simulink model "spaceShuttleOriginal"  (R2017b)
settings: Solver=FixedStepAuto  StartTime=0.0  StopTime=300  FixedStep=0.08  RelTol=1e-3
undefined symbols (not defined in the file or in its folder): ATTITUDE_ESTIMATE, ATTITUDE_INCREMENT, AUTO_MANUAL_SWITCH, BYPASS, COUNTER, CURRENT_ATTITUDE, DESIRED_ATTITUDE, DESIRED_RATE, INIT_AUTO_MANEUVER, INIT_JET_SELECT, INIT_STATE_ERROR, MANEUVER_HOLD_SW, PRIMARY_JET_COMMAND, RATE_ESTIMATE, UNDESIRED_ACCELERATION_ESTIMATE, VERNIER_JET_COMMAND
libraries: sharedtransform x5, aerolibutil x4, realtime_pacer_lib x1
(part 1 of 3)
settings Model: Creator=raphael  LastModifiedBy=hbourbou

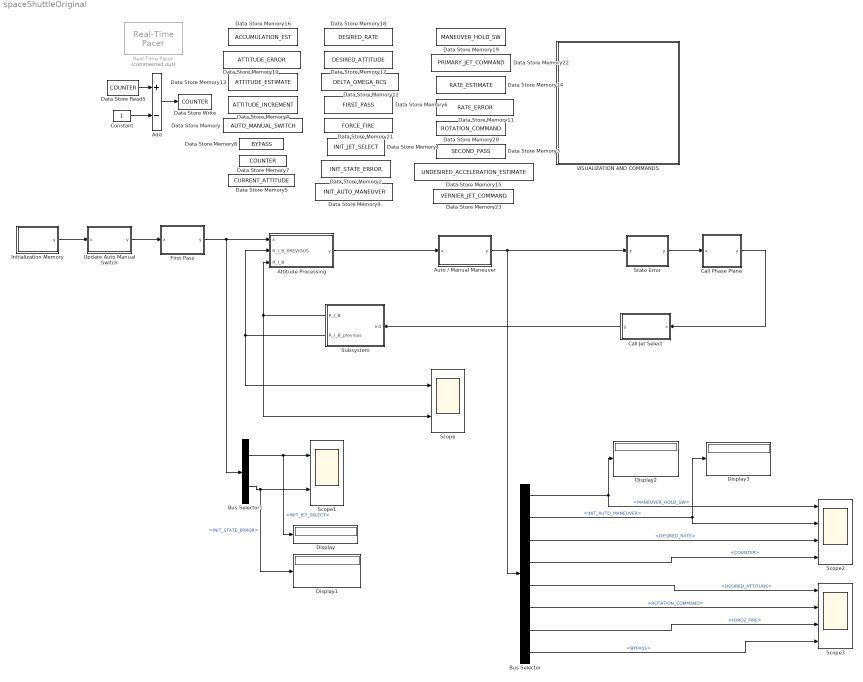
== system spaceShuttleOriginal ==
  Add : Sum  Inputs=+-
  Attitude Processing : Subsystem  Priority=2
  Auto / Manual Maneuver : Subsystem  Priority=2
  Bus Selector : BusSelector  OutputSignals=MANEUVER_HOLD_SW,INIT_AUTO_MANEUVER,DESIRED_RATE,COUNTER,DESIRED_ATTITUDE,ROTATION_COMMAND,FORCE_FIRE,BYPASS
  Bus Selector1 : BusSelector  OutputSignals=INIT_JET_SELECT,INIT_STATE_ERROR
  Call Jet Select : Subsystem  Priority=2
  Call Phase Plane : Subsystem  Priority=2
  Constant : Constant  SampleTime=-1
  Data Store Memory : DataStoreMemory  DataStoreName=AUTO_MANUAL_SWITCH  ReadBeforeWriteMsg=warning  WriteAfterWriteMsg=warning  WriteAfterReadMsg=warning  InitialValue=[0;0]  ShowAdditionalParam=off
  Data Store Memory1 : DataStoreMemory  DataStoreName=INIT_JET_SELECT  ReadBeforeWriteMsg=warning  WriteAfterWriteMsg=warning  WriteAfterReadMsg=warning  ShowAdditionalParam=off
  Data Store Memory10 : DataStoreMemory  DataStoreName=ATTITUDE_ERROR  ReadBeforeWriteMsg=warning  WriteAfterWriteMsg=warning  WriteAfterReadMsg=warning  InitialValue=[0;0;0]  ShowAdditionalParam=off  Dimensions=3
  Data Store Memory11 : DataStoreMemory  DataStoreName=RATE_ERROR  ReadBeforeWriteMsg=warning  WriteAfterWriteMsg=warning  WriteAfterReadMsg=warning  InitialValue=[0;0;0]  ShowAdditionalParam=off  Dimensions=3
  Data Store Memory12 : DataStoreMemory  DataStoreName=DELTA_OMEGA_RCS  ReadBeforeWriteMsg=warning  WriteAfterWriteMsg=warning  WriteAfterReadMsg=warning  InitialValue=[0;0;0]  ShowAdditionalParam=off  Dimensions=3
  Data Store Memory13 : DataStoreMemory  DataStoreName=ATTITUDE_ESTIMATE  ReadBeforeWriteMsg=warning  WriteAfterWriteMsg=warning  WriteAfterReadMsg=warning  InitialValue=[0;0;0]  ShowAdditionalParam=off  Dimensions=3
  Data Store Memory14 : DataStoreMemory  DataStoreName=RATE_ESTIMATE  ReadBeforeWriteMsg=warning  WriteAfterWriteMsg=warning  WriteAfterReadMsg=warning  InitialValue=[0;0;0]  ShowAdditionalParam=off  Dimensions=3
  Data Store Memory15 : DataStoreMemory  DataStoreName=UNDESIRED_ACCELERATION_ESTIMATE  ReadBeforeWriteMsg=warning  WriteAfterWriteMsg=warning  WriteAfterReadMsg=warning  InitialValue=[0;0;0]  ShowAdditionalParam=off  Dimensions=3
  Data Store Memory16 : DataStoreMemory  DataStoreName=ACCUMULATION_EST  ReadBeforeWriteMsg=warning  WriteAfterWriteMsg=warning  WriteAfterReadMsg=warning  InitialValue=[0;0;0]  ShowAdditionalParam=off  Dimensions=3
  Data Store Memory17 : DataStoreMemory  DataStoreName=DESIRED_ATTITUDE  ReadBeforeWriteMsg=warning  WriteAfterWriteMsg=warning  WriteAfterReadMsg=warning  InitialValue=[0;0;0]  ShowAdditionalParam=off  Dimensions=3
  Data Store Memory18 : DataStoreMemory  DataStoreName=DESIRED_RATE  ReadBeforeWriteMsg=warning  WriteAfterWriteMsg=warning  WriteAfterReadMsg=warning  InitialValue=[0;0;0]  ShowAdditionalParam=off  Dimensions=3
  Data Store Memory19 : DataStoreMemory  DataStoreName=MANEUVER_HOLD_SW  ReadBeforeWriteMsg=warning  WriteAfterWriteMsg=warning  WriteAfterReadMsg=warning  InitialValue=[0;0]  ShowAdditionalParam=off  Dimensions=2
  Data Store Memory2 : DataStoreMemory  DataStoreName=INIT_STATE_ERROR  ReadBeforeWriteMsg=warning  WriteAfterWriteMsg=warning  WriteAfterReadMsg=warning  InitialValue=[0;0;0]  ShowAdditionalParam=off  Dimensions=3
  Data Store Memory20 : DataStoreMemory  DataStoreName=ROTATION_COMMAND  ReadBeforeWriteMsg=warning  WriteAfterWriteMsg=warning  WriteAfterReadMsg=warning  InitialValue=[0;0;0]  ShowAdditionalParam=off  Dimensions=3
  Data Store Memory21 : DataStoreMemory  DataStoreName=FORCE_FIRE  ReadBeforeWriteMsg=warning  WriteAfterWriteMsg=warning  WriteAfterReadMsg=warning  InitialValue=[0;0;0]  ShowAdditionalParam=off  Dimensions=3
  Data Store Memory22 : DataStoreMemory  DataStoreName=PRIMARY_JET_COMMAND  ReadBeforeWriteMsg=warning  WriteAfterWriteMsg=warning  WriteAfterReadMsg=warning  InitialValue=[0;0;0;0;0;0;0;0;0;0;0]  ShowAdditionalParam=off  Dimensions=11
  Data Store Memory23 : DataStoreMemory  DataStoreName=VERNIER_JET_COMMAND  ReadBeforeWriteMsg=warning  WriteAfterWriteMsg=warning  WriteAfterReadMsg=warning  InitialValue=[0;0;0;0;0;0]  ShowAdditionalParam=off  Dimensions=6
  Data Store Memory3 : DataStoreMemory  DataStoreName=SECOND_PASS  ReadBeforeWriteMsg=warning  WriteAfterWriteMsg=warning  WriteAfterReadMsg=warning  ShowAdditionalParam=off
  Data Store Memory4 : DataStoreMemory  DataStoreName=ATTITUDE_INCREMENT  ReadBeforeWriteMsg=warning  WriteAfterWriteMsg=warning  WriteAfterReadMsg=warning  InitialValue=[0;0;0]  ShowAdditionalParam=off  Dimensions=3
  Data Store Memory5 : DataStoreMemory  DataStoreName=CURRENT_ATTITUDE  ReadBeforeWriteMsg=warning  WriteAfterWriteMsg=warning  WriteAfterReadMsg=warning  InitialValue=[0;0;0;0]  ShowAdditionalParam=off  Dimensions=4
  Data Store Memory6 : DataStoreMemory  DataStoreName=FIRST_PASS  ReadBeforeWriteMsg=warning  WriteAfterWriteMsg=warning  WriteAfterReadMsg=warning  InitialValue=1  ShowAdditionalParam=off  Dimensions=1
  Data Store Memory7 : DataStoreMemory  DataStoreName=COUNTER  ReadBeforeWriteMsg=warning  WriteAfterWriteMsg=warning  WriteAfterReadMsg=warning  ShowAdditionalParam=off  Dimensions=1
  Data Store Memory8 : DataStoreMemory  DataStoreName=BYPASS  ReadBeforeWriteMsg=warning  WriteAfterWriteMsg=warning  WriteAfterReadMsg=warning  InitialValue=[1;1;1]  ShowAdditionalParam=off  Dimensions=3
  Data Store Memory9 : DataStoreMemory  DataStoreName=INIT_AUTO_MANEUVER  ReadBeforeWriteMsg=warning  WriteAfterWriteMsg=warning  WriteAfterReadMsg=warning  InitialValue=[0]  ShowAdditionalParam=off  Dimensions=1
  Data Store Read5 : DataStoreRead  DataStoreName=COUNTER
  Data Store Write : DataStoreWrite  DataStoreName=COUNTER
  Display{,1..3} (4 alike) : Display
  First Pass : Subsystem  Priority=2
  Initialization Memory : Subsystem
  Real-Time Pacer : realtime_pacer_lib/Real-Time Pacer  Commented=on  simTimePerRealTime=1
  Scope : Scope  NumInputPorts=2
  Scope1 : Scope  NumInputPorts=2
  Scope2 : Scope  NumInputPorts=4
  Scope3 : Scope  NumInputPorts=4
  State Error : Subsystem  Priority=2
  Subsystem : Subsystem
      mask Display: image(imread('spaceShuttle.jpg','jpg'),'center')
  Update Auto Manual Switch : Subsystem  Priority=2
  VISUALIZATION AND COMMANDS : Subsystem
  wires:
  Update Auto Manual Switch/1(y) -> First Pass/1(x)
  First Pass/1(y) -> Bus Selector1/1, Attitude Processing/1(x)
  Data Store Read5/1 -> Add/1
  Constant/1 -> Add/2
  Add/1 -> Data Store Write/1
  Attitude Processing/1(y) -> Auto / Manual Maneuver/1(x)
  Auto / Manual Maneuver/1(y) -> Bus Selector/1, State Error/1(x)
  State Error/1(y) -> Call Phase Plane/1(x)
  Call Phase Plane/1(y) -> Call Jet Select/1(x)
  Call Jet Select/1(y) -> Subsystem/1(In1)
  Subsystem/1(R_I_B) -> Attitude Processing/3(R_I_B), Scope/2
  Subsystem/2(R_I_B_previous) -> Attitude Processing/2(R_I_B_PREVIOUS), Scope/1
  Initialization Memory/1(y) -> Update Auto Manual Switch/1(x)
  Bus Selector/1 -> Display2/1, Scope2/1  "<MANEUVER_HOLD_SW>"
  Bus Selector/2 -> Display3/1, Scope2/2  "<INIT_AUTO_MANEUVER>"
  Bus Selector/3 -> Scope2/3  "<DESIRED_RATE>"
  Bus Selector/4 -> Scope2/4  "<COUNTER>"
  Bus Selector1/1 -> Display/1, Scope1/1  "<INIT_JET_SELECT>"
  Bus Selector1/2 -> Display1/1, Scope1/2  "<INIT_STATE_ERROR>"
  Bus Selector/5 -> Scope3/1  "<DESIRED_ATTITUDE>"
  Bus Selector/6 -> Scope3/2  "<ROTATION_COMMAND>"
  Bus Selector/7 -> Scope3/3  "<FORCE_FIRE>"
  Bus Selector/8 -> Scope3/4  "<BYPASS>"

== system spaceShuttleOriginal/Attitude Processing ==
  x : Inport
  R_I_B_PREVIOUS : Inport  Port=2
  R_I_B : Inport  Port=3
  Data Store Read : DataStoreRead  DataStoreName=SECOND_PASS
  If : If  IfExpression=u1 == 1
  Merge : Merge
  SECOND_PASS == 0 : Subsystem  TreatAsAtomicUnit=on
  SECOND_PASS == 1 : Subsystem  TreatAsAtomicUnit=on
  y : Outport
  wires:
  x/1 -> SECOND_PASS == 0/1(x), SECOND_PASS == 1/1(x)
  Data Store Read/1 -> If/1
  SECOND_PASS == 1/1(y) -> Merge/1
  If/1 -> SECOND_PASS == 1/Action
  If/2 -> SECOND_PASS == 0/Action
  SECOND_PASS == 0/1(y) -> Merge/2
  Merge/1 -> y/1
  R_I_B/1 -> SECOND_PASS == 1/2(R_I_B)
  R_I_B_PREVIOUS/1 -> SECOND_PASS == 1/3(R_I_B1)

== system spaceShuttleOriginal/Auto // Manual Maneuver ==
  x : Inport
  Bus Selector1 : BusSelector  OutputSignals=AUTO_MANUAL_SWITCH
  IF MANUAL : Subsystem  TreatAsAtomicUnit=on
  If : If  IfExpression=u1 == 1
  If AUTO : Subsystem  TreatAsAtomicUnit=on
  Merge : Merge
  Selector : Selector  InputPortWidth=2  IndexOptions=Index vector (dialog)  Indices=[1]  OutputSizes=1
  y : Outport
  wires:
  Selector/1 -> If/1
  If/1 -> If AUTO/Action
  Bus Selector1/1 -> Selector/1  "<AUTO_MANUAL_SWITCH>"
  x/1 -> IF MANUAL/1(x), If AUTO/1(x), Bus Selector1/1
  If/2 -> IF MANUAL/Action
  Merge/1 -> y/1
  IF MANUAL/1(y) -> Merge/2
  If AUTO/1(Out1) -> Merge/1

== system spaceShuttleOriginal/Call Jet Select ==
  x : Inport
  Bus Assignment : BusAssignment  AssignedSignals=INIT_JET_SELECT
  Bus Selector1 : BusSelector  OutputSignals=USER_INPUTS.PRIMARY_VERNIER_SW
  Constant2 : Constant  Value=0
  Data Store Write : DataStoreWrite  DataStoreName=INIT_JET_SELECT
  If : If  IfExpression=u1 == 1
  Merge : Merge
  PRIMARY JETS : Subsystem  TreatAsAtomicUnit=on
  VERNIER JETS : Subsystem  TreatAsAtomicUnit=on
  y : Outport
  wires:
  x/1 -> VERNIER JETS/1(x), PRIMARY JETS/1(In1), Bus Selector1/1
  If/1 -> PRIMARY JETS/Action
  PRIMARY JETS/1(y) -> Merge/1
  If/2 -> VERNIER JETS/Action
  Bus Selector1/1 -> If/1  "<PRIMARY_VERNIER_SW>"
  VERNIER JETS/1(y) -> Merge/2
  Constant2/1 -> Bus Assignment/2, Data Store Write/1
  Merge/1 -> Bus Assignment/1
  Bus Assignment/1 -> y/1

== system spaceShuttleOriginal/Call Phase Plane ==
  x : Inport
  Bus Assignment : BusAssignment  AssignedSignals=ROTATION_COMMAND
  Data Store Write : DataStoreWrite  DataStoreName=ROTATION_COMMAND
  Display : Display
  Get Rotation Pitch : Subsystem
  Get Rotation Roll : Subsystem
  Get Rotation Yaw : Subsystem
  Mux : Mux  Inputs=3
  y : Outport
  wires:
  x/1 -> Get Rotation Roll/1(In1), Bus Assignment/1, Get Rotation Yaw/1(In1), Get Rotation Pitch/1(In1)
  Get Rotation Yaw/1(Out1) -> Mux/3
  Mux/1 -> Display/1, Data Store Write/1, Bus Assignment/2
  Get Rotation Roll/1(Out1) -> Mux/1
  Get Rotation Pitch/1(Out1) -> Mux/2
  Bus Assignment/1 -> y/1

== system spaceShuttleOriginal/First Pass ==
  x : Inport
  Bus Selector : BusSelector  OutputSignals=FIRST_PASS
  If : If  IfExpression=u1 == 1
  If First Pass : Subsystem  TreatAsAtomicUnit=on
  If not first pass : Subsystem  TreatAsAtomicUnit=on
  Merge : Merge
  y : Outport
  wires:
  x/1 -> If not first pass/1(In1), Bus Selector/1, If First Pass/1(In1)
  If not first pass/1(x) -> Merge/2
  If/1 -> If First Pass/Action
  If/2 -> If not first pass/Action
  If First Pass/1(x) -> Merge/1
  Merge/1 -> y/1
  Bus Selector/1 -> If/1  "<FIRST_PASS>"

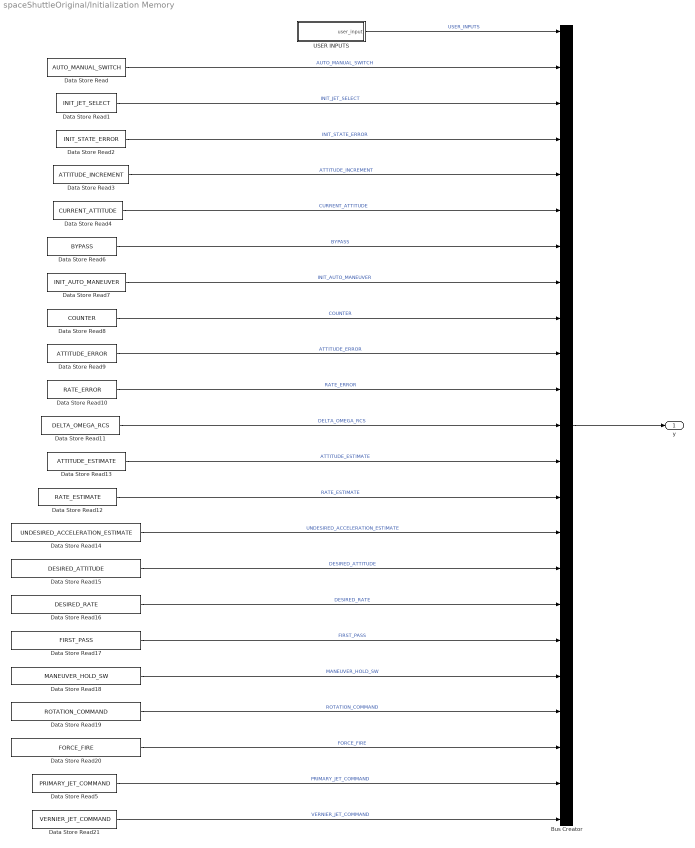
== system spaceShuttleOriginal/Initialization Memory ==
  Bus Creator : BusCreator  Inputs=23
  Data Store Read : DataStoreRead  DataStoreName=AUTO_MANUAL_SWITCH
  Data Store Read1 : DataStoreRead  DataStoreName=INIT_JET_SELECT
  Data Store Read10 : DataStoreRead  DataStoreName=RATE_ERROR
  Data Store Read11 : DataStoreRead  DataStoreName=DELTA_OMEGA_RCS
  Data Store Read12 : DataStoreRead  DataStoreName=RATE_ESTIMATE
  Data Store Read13 : DataStoreRead  DataStoreName=ATTITUDE_ESTIMATE
  Data Store Read14 : DataStoreRead  DataStoreName=UNDESIRED_ACCELERATION_ESTIMATE
  Data Store Read15 : DataStoreRead  DataStoreName=DESIRED_ATTITUDE
  Data Store Read16 : DataStoreRead  DataStoreName=DESIRED_RATE
  Data Store Read17 : DataStoreRead  DataStoreName=FIRST_PASS
  Data Store Read18 : DataStoreRead  DataStoreName=MANEUVER_HOLD_SW
  Data Store Read19 : DataStoreRead  DataStoreName=ROTATION_COMMAND
  Data Store Read2 : DataStoreRead  DataStoreName=INIT_STATE_ERROR
  Data Store Read20 : DataStoreRead  DataStoreName=FORCE_FIRE
  Data Store Read21 : DataStoreRead  DataStoreName=VERNIER_JET_COMMAND
  Data Store Read3 : DataStoreRead  DataStoreName=ATTITUDE_INCREMENT
  Data Store Read4 : DataStoreRead  DataStoreName=CURRENT_ATTITUDE
  Data Store Read5 : DataStoreRead  DataStoreName=PRIMARY_JET_COMMAND
  Data Store Read6 : DataStoreRead  DataStoreName=BYPASS
  Data Store Read7 : DataStoreRead  DataStoreName=INIT_AUTO_MANEUVER
  Data Store Read8 : DataStoreRead  DataStoreName=COUNTER
  Data Store Read9 : DataStoreRead  DataStoreName=ATTITUDE_ERROR
  USER INPUTS : Subsystem  Priority=1
  y : Outport
  wires:
  Data Store Read/1 -> Bus Creator/2  "AUTO_MANUAL_SWITCH"
  Data Store Read1/1 -> Bus Creator/3  "INIT_JET_SELECT"
  Data Store Read2/1 -> Bus Creator/4  "INIT_STATE_ERROR"
  Data Store Read3/1 -> Bus Creator/5  "ATTITUDE_INCREMENT"
  Data Store Read4/1 -> Bus Creator/6  "CURRENT_ATTITUDE"
  Data Store Read6/1 -> Bus Creator/7  "BYPASS"
  Data Store Read7/1 -> Bus Creator/8  "INIT_AUTO_MANEUVER"
  Data Store Read8/1 -> Bus Creator/9  "COUNTER"
  Data Store Read9/1 -> Bus Creator/10  "ATTITUDE_ERROR"
  Data Store Read10/1 -> Bus Creator/11  "RATE_ERROR"
  Data Store Read11/1 -> Bus Creator/12  "DELTA_OMEGA_RCS"
  Data Store Read14/1 -> Bus Creator/15  "UNDESIRED_ACCELERATION_ESTIMATE"
  Data Store Read13/1 -> Bus Creator/13  "ATTITUDE_ESTIMATE"
  Data Store Read12/1 -> Bus Creator/14  "RATE_ESTIMATE"
  Data Store Read15/1 -> Bus Creator/16  "DESIRED_ATTITUDE"
  Data Store Read16/1 -> Bus Creator/17  "DESIRED_RATE"
  Data Store Read17/1 -> Bus Creator/18  "FIRST_PASS"
  Bus Creator/1 -> y/1
  Data Store Read18/1 -> Bus Creator/19  "MANEUVER_HOLD_SW"
  Data Store Read19/1 -> Bus Creator/20  "ROTATION_COMMAND"
  Data Store Read20/1 -> Bus Creator/21  "FORCE_FIRE"
  Data Store Read5/1 -> Bus Creator/22  "PRIMARY_JET_COMMAND"
  USER INPUTS/1(user_input) -> Bus Creator/1  "USER_INPUTS"
  Data Store Read21/1 -> Bus Creator/23  "VERNIER_JET_COMMAND"

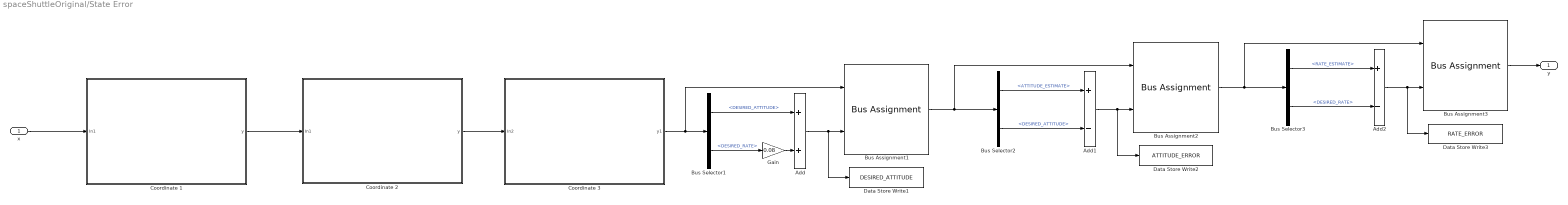
== system spaceShuttleOriginal/State Error ==
  x : Inport
  Add : Sum
  Add1 : Sum  Inputs=+-
  Add2 : Sum  Inputs=+-
  Bus Assignment1 : BusAssignment  AssignedSignals=DESIRED_ATTITUDE
  Bus Assignment2 : BusAssignment  AssignedSignals=ATTITUDE_ERROR
  Bus Assignment3 : BusAssignment  AssignedSignals=RATE_ERROR
  Bus Selector1 : BusSelector  OutputSignals=DESIRED_ATTITUDE,DESIRED_RATE
  Bus Selector2 : BusSelector  OutputSignals=ATTITUDE_ESTIMATE,DESIRED_ATTITUDE
  Bus Selector3 : BusSelector  OutputSignals=RATE_ESTIMATE,DESIRED_RATE
  Coordinate 1 : Subsystem
  Coordinate 2 : Subsystem
  Coordinate 3 : Subsystem
  Data Store Write1 : DataStoreWrite  DataStoreName=DESIRED_ATTITUDE
  Data Store Write2 : DataStoreWrite  DataStoreName=ATTITUDE_ERROR
  Data Store Write3 : DataStoreWrite  DataStoreName=RATE_ERROR
  Gain : Gain  Gain=0.08
  y : Outport
  wires:
  x/1 -> Coordinate 1/1(In1)
  Coordinate 2/1(y) -> Coordinate 3/1(In2)
  Coordinate 1/1(y) -> Coordinate 2/1(In1)
  Bus Assignment1/1 -> Bus Assignment2/1, Bus Selector2/1
  Gain/1 -> Add/2
  Bus Selector2/2 -> Add1/2  "<DESIRED_ATTITUDE>"
  Bus Selector1/1 -> Add/1  "<DESIRED_ATTITUDE>"
  Bus Selector2/1 -> Add1/1  "<ATTITUDE_ESTIMATE>"
  Bus Selector3/2 -> Add2/2  "<DESIRED_RATE>"
  Add1/1 -> Bus Assignment2/2, Data Store Write2/1
  Bus Selector3/1 -> Add2/1  "<RATE_ESTIMATE>"
  Bus Assignment2/1 -> Bus Assignment3/1, Bus Selector3/1
  Bus Assignment3/1 -> y/1
  Add/1 -> Bus Assignment1/2, Data Store Write1/1
  Bus Selector1/2 -> Gain/1  "<DESIRED_RATE>"
  Coordinate 3/1(y1) -> Bus Selector1/1, Bus Assignment1/1
  Add2/1 -> Bus Assignment3/2, Data Store Write3/1

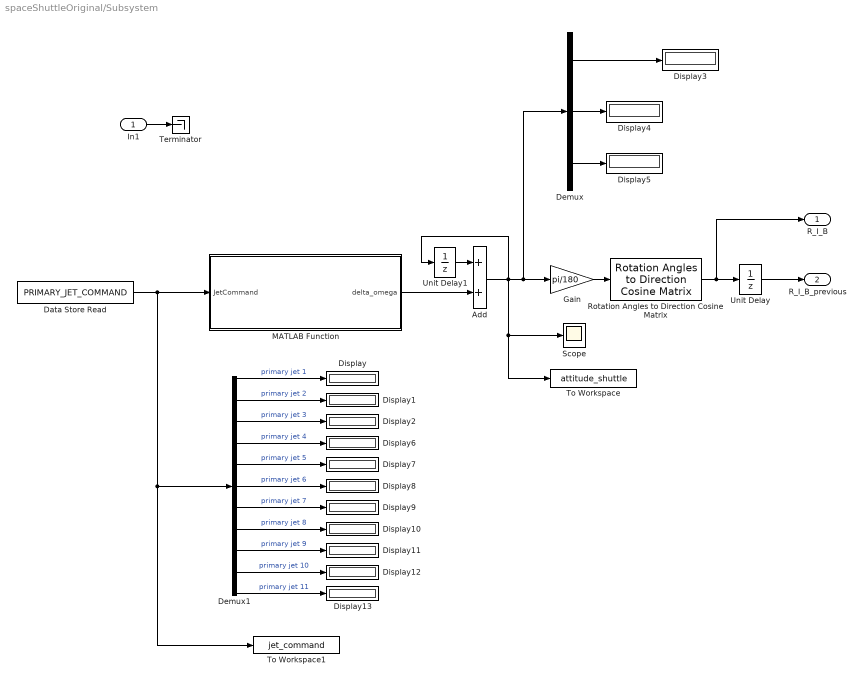
== system spaceShuttleOriginal/Subsystem ==
  In1 : Inport
  Add : Sum
  Data Store Read : DataStoreRead  DataStoreName=PRIMARY_JET_COMMAND
  Demux : Demux  Outputs=3
  Demux1 : Demux  Outputs=11
  Display{,1..13} (14 alike) : Display
  Gain : Gain  Gain=pi/180
  MATLAB Function : MATLAB Function  TreatAsAtomicUnit=on
  Rotation Angles to Direction Cosine Matrix : sharedtransform/Rotation Angles to Direction Cosine Matrix  rotationOrder=XYZ
      settings: SourceProductBaseCode=AE
  Scope : Scope
  Terminator : Terminator
  To Workspace : ToWorkspace  VariableName=attitude_shuttle  SaveFormat=Timeseries  SampleTime=-1
  To Workspace1 : ToWorkspace  VariableName=jet_command  SaveFormat=Timeseries  SampleTime=-1
  Unit Delay : UnitDelay  InitialCondition=eye(3)  SampleTime=-1
  Unit Delay1 : UnitDelay  InitialCondition=[50;50;50]  SampleTime=-1
  R_I_B : Outport
  R_I_B_previous : Outport  Port=2
  wires:
  Gain/1 -> Rotation Angles to Direction Cosine Matrix/1
  Unit Delay1/1 -> Add/1
  Add/1 -> Gain/1, Demux/1, To Workspace/1, Scope/1, Unit Delay1/1
  MATLAB Function/1(delta_omega) -> Add/2
  Demux/3 -> Display5/1
  Demux/2 -> Display4/1
  Demux/1 -> Display3/1
  Demux1/1 -> Display/1  "primary jet 1"
  Demux1/2 -> Display1/1  "primary jet 2"
  Demux1/7 -> Display9/1  "primary jet 7"
  Demux1/6 -> Display8/1  "primary jet 6"
  Demux1/5 -> Display7/1  "primary jet 5"
  Demux1/4 -> Display6/1  "primary jet 4"
  Demux1/3 -> Display2/1  "primary jet 3"
  Demux1/9 -> Display11/1  "primary jet 9"
  Demux1/8 -> Display10/1  "primary jet 8"
  Demux1/10 -> Display12/1  "primary jet 10"
  Demux1/11 -> Display13/1  "primary jet 11"
  Unit Delay/1 -> R_I_B_previous/1
  Rotation Angles to Direction Cosine Matrix/1 -> R_I_B/1, Unit Delay/1
  In1/1 -> Terminator/1
  Data Store Read/1 -> Demux1/1, To Workspace1/1, MATLAB Function/1(JetCommand)

== system spaceShuttleOriginal/Update Auto Manual Switch ==
  x : Inport
  Bus Selector : BusSelector  OutputSignals=RHC_STATE
  Bus Selector1 : BusSelector  OutputSignals=USER_INPUTS
  Dot Product : DotProduct  InputSameDT=on  OutDataTypeStr=Inherit: Inherit via internal rule
  IF RHC : Subsystem  TreatAsAtomicUnit=on
  If : If  IfExpression=u1 ~= 0
  Merge : Merge
  NO RHC : Subsystem  TreatAsAtomicUnit=on
  Sqrt : Sqrt  SaturateOnIntegerOverflow=on
  y : Outport
  wires:
  Dot Product/1 -> Sqrt/1
  If/1 -> IF RHC/Action
  x/1 -> Bus Selector1/1, IF RHC/1(In1), NO RHC/1(In1)
  Bus Selector/1 -> Dot Product/1, Dot Product/2  "<RHC_STATE>"
  If/2 -> NO RHC/Action
  IF RHC/1(x) -> Merge/1
  NO RHC/1(x1) -> Merge/2
  Merge/1 -> y/1
  Sqrt/1 -> If/1
  Bus Selector1/1 -> Bus Selector/1  "<USER_INPUTS>"

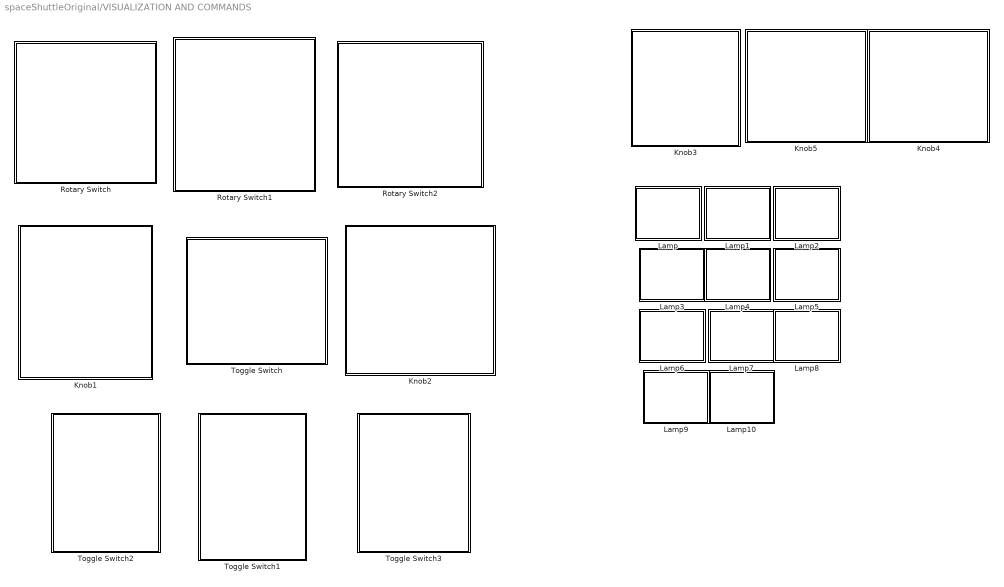
== system spaceShuttleOriginal/VISUALIZATION AND COMMANDS ==
  Knob1 : Subsystem  DialogController=hmiCreateDDGDialog  IsWebBlock=on  mask(MWDashboardBlock){webBlockId=fcc256ec-b885-471c-9536-edbe70c05013, webBlockType=continuousknob, ShowInLibBrowser=on, ShowInitialText=on, HMISrcModelName=spaceShuttleOriginal}
      mask prompts: webBlockId "WebBlock Id"; webBlockType "WebBlock Type"; HMISrcModelName "Source Model"
      mask help: SimulinkHMI:dialogs:ContinuousKnobDialogDesc
      mask Help: helpview([docroot '/mapfiles/simulink.map'], 'hmi_knob')
      mask Display:
      | if strcmp(get_param(bdroot(gcb),'BlockDiagramType'), 'library')
      |     image([(matlabroot) '/toolbox/simulink/hmi/icons/ContinuousKnob.png']);
      | end
  Knob2 : Subsystem  DialogController=hmiCreateDDGDialog  IsWebBlock=on  mask(MWDashboardBlock){webBlockId=8f75210b-2a30-49d8-9c3f-54d330528343, webBlockType=continuousknob, ShowInLibBrowser=on, ShowInitialText=on, HMISrcModelName=spaceShuttleOriginal}
      mask prompts: webBlockId "WebBlock Id"; webBlockType "WebBlock Type"; HMISrcModelName "Source Model"
      mask help: SimulinkHMI:dialogs:ContinuousKnobDialogDesc
      mask Help: helpview([docroot '/mapfiles/simulink.map'], 'hmi_knob')
      mask Display:
      | if strcmp(get_param(bdroot(gcb),'BlockDiagramType'), 'library')
      |     image([(matlabroot) '/toolbox/simulink/hmi/icons/ContinuousKnob.png']);
      | end
  Knob3 : Subsystem  DialogController=hmiCreateDDGDialog  IsWebBlock=on  mask(MWDashboardBlock){webBlockId=1d9576ac-1a07-4627-a000-52538d07e885, webBlockType=continuousknob, ShowInLibBrowser=on, ShowInitialText=on, HMISrcModelName=spaceShuttleOriginal}
      mask prompts: webBlockId "WebBlock Id"; webBlockType "WebBlock Type"; HMISrcModelName "Source Model"
      mask help: SimulinkHMI:dialogs:ContinuousKnobDialogDesc
      mask Help: helpview([docroot '/mapfiles/simulink.map'], 'hmi_knob')
      mask Display:
      | if strcmp(get_param(bdroot(gcb),'BlockDiagramType'), 'library')
      |     image([(matlabroot) '/toolbox/simulink/hmi/icons/ContinuousKnob.png']);
      | end
  Knob4 : Subsystem  DialogController=hmiCreateDDGDialog  IsWebBlock=on  mask(MWDashboardBlock){webBlockId=ba6a8299-7a60-4fd1-b3c4-837f140646ce, webBlockType=continuousknob, ShowInLibBrowser=on, ShowInitialText=on, HMISrcModelName=spaceShuttleOriginal}
      mask prompts: webBlockId "WebBlock Id"; webBlockType "WebBlock Type"; HMISrcModelName "Source Model"
      mask help: SimulinkHMI:dialogs:ContinuousKnobDialogDesc
      mask Help: helpview([docroot '/mapfiles/simulink.map'], 'hmi_knob')
      mask Display:
      | if strcmp(get_param(bdroot(gcb),'BlockDiagramType'), 'library')
      |     image([(matlabroot) '/toolbox/simulink/hmi/icons/ContinuousKnob.png']);
      | end
  Knob5 : Subsystem  DialogController=hmiCreateDDGDialog  IsWebBlock=on  mask(MWDashboardBlock){webBlockId=36d52b40-e662-4d56-9627-14147bf9ee74, webBlockType=continuousknob, ShowInLibBrowser=on, ShowInitialText=on, HMISrcModelName=spaceShuttleOriginal}
      mask prompts: webBlockId "WebBlock Id"; webBlockType "WebBlock Type"; HMISrcModelName "Source Model"
      mask help: SimulinkHMI:dialogs:ContinuousKnobDialogDesc
      mask Help: helpview([docroot '/mapfiles/simulink.map'], 'hmi_knob')
      mask Display:
      | if strcmp(get_param(bdroot(gcb),'BlockDiagramType'), 'library')
      |     image([(matlabroot) '/toolbox/simulink/hmi/icons/ContinuousKnob.png']);
      | end
  Lamp : Subsystem  DialogController=hmiCreateDDGDialog  IsWebBlock=on  mask(MWDashboardBlock){webBlockId=1831b2f3-6b24-4792-bd35-9106f5a9402c, webBlockType=lamp, ShowInLibBrowser=on, ShowInitialText=on, HMISrcModelName=spaceShuttleOriginal}
      mask prompts: webBlockType "WebBlock Type"; HMISrcModelName "Source Model"
      mask help: SimulinkHMI:dialogs:LampDialogDesc
      mask Help: helpview([docroot '/mapfiles/simulink.map'], 'hmi_lamp')
      mask Display:
      | if strcmp(get_param(bdroot(gcb),'BlockDiagramType'), 'library')
      |     image([(matlabroot) '/toolbox/simulink/hmi/icons/Lamp.png']);
      | end
  Lamp1 : Subsystem  DialogController=hmiCreateDDGDialog  IsWebBlock=on  mask(MWDashboardBlock){webBlockId=445b80d1-ef4e-4a60-adf9-cfd209c84993, webBlockType=lamp, ShowInLibBrowser=on, ShowInitialText=on, HMISrcModelName=spaceShuttleOriginal}
      mask prompts: webBlockType "WebBlock Type"; HMISrcModelName "Source Model"
      mask help: SimulinkHMI:dialogs:LampDialogDesc
      mask Help: helpview([docroot '/mapfiles/simulink.map'], 'hmi_lamp')
      mask Display:
      | if strcmp(get_param(bdroot(gcb),'BlockDiagramType'), 'library')
      |     image([(matlabroot) '/toolbox/simulink/hmi/icons/Lamp.png']);
      | end
  Lamp10 : Subsystem  DialogController=hmiCreateDDGDialog  IsWebBlock=on  mask(MWDashboardBlock){webBlockId=5e79d13d-1851-4c1d-ad64-373adbe08a7d, webBlockType=lamp, ShowInLibBrowser=on, ShowInitialText=on, HMISrcModelName=spaceShuttleOriginal}
      mask prompts: webBlockType "WebBlock Type"; HMISrcModelName "Source Model"
      mask help: SimulinkHMI:dialogs:LampDialogDesc
      mask Help: helpview([docroot '/mapfiles/simulink.map'], 'hmi_lamp')
      mask Display:
      | if strcmp(get_param(bdroot(gcb),'BlockDiagramType'), 'library')
      |     image([(matlabroot) '/toolbox/simulink/hmi/icons/Lamp.png']);
      | end
  Lamp2 : Subsystem  DialogController=hmiCreateDDGDialog  IsWebBlock=on  mask(MWDashboardBlock){webBlockId=fe722917-839e-4c17-b303-c27dc3d815a5, webBlockType=lamp, ShowInLibBrowser=on, ShowInitialText=on, HMISrcModelName=spaceShuttleOriginal}
      mask prompts: webBlockType "WebBlock Type"; HMISrcModelName "Source Model"
      mask help: SimulinkHMI:dialogs:LampDialogDesc
      mask Help: helpview([docroot '/mapfiles/simulink.map'], 'hmi_lamp')
      mask Display:
      | if strcmp(get_param(bdroot(gcb),'BlockDiagramType'), 'library')
      |     image([(matlabroot) '/toolbox/simulink/hmi/icons/Lamp.png']);
      | end
  Lamp3 : Subsystem  DialogController=hmiCreateDDGDialog  IsWebBlock=on  mask(MWDashboardBlock){webBlockId=892c30e5-c3e8-4f09-b059-7bca243d068a, webBlockType=lamp, ShowInLibBrowser=on, ShowInitialText=on, HMISrcModelName=spaceShuttleOriginal}
      mask prompts: webBlockType "WebBlock Type"; HMISrcModelName "Source Model"
      mask help: SimulinkHMI:dialogs:LampDialogDesc
      mask Help: helpview([docroot '/mapfiles/simulink.map'], 'hmi_lamp')
      mask Display:
      | if strcmp(get_param(bdroot(gcb),'BlockDiagramType'), 'library')
      |     image([(matlabroot) '/toolbox/simulink/hmi/icons/Lamp.png']);
      | end
  Lamp4 : Subsystem  DialogController=hmiCreateDDGDialog  IsWebBlock=on  mask(MWDashboardBlock){webBlockId=c806c832-793b-4743-9fcd-4b551699f67b, webBlockType=lamp, ShowInLibBrowser=on, ShowInitialText=on, HMISrcModelName=spaceShuttleOriginal}
      mask prompts: webBlockType "WebBlock Type"; HMISrcModelName "Source Model"
      mask help: SimulinkHMI:dialogs:LampDialogDesc
      mask Help: helpview([docroot '/mapfiles/simulink.map'], 'hmi_lamp')
      mask Display:
      | if strcmp(get_param(bdroot(gcb),'BlockDiagramType'), 'library')
      |     image([(matlabroot) '/toolbox/simulink/hmi/icons/Lamp.png']);
      | end
  Lamp5 : Subsystem  DialogController=hmiCreateDDGDialog  IsWebBlock=on  mask(MWDashboardBlock){webBlockId=98e8761d-c632-4f86-92e2-3e19c3b791e9, webBlockType=lamp, ShowInLibBrowser=on, ShowInitialText=on, HMISrcModelName=spaceShuttleOriginal}
      mask prompts: webBlockType "WebBlock Type"; HMISrcModelName "Source Model"
      mask help: SimulinkHMI:dialogs:LampDialogDesc
      mask Help: helpview([docroot '/mapfiles/simulink.map'], 'hmi_lamp')
      mask Display:
      | if strcmp(get_param(bdroot(gcb),'BlockDiagramType'), 'library')
      |     image([(matlabroot) '/toolbox/simulink/hmi/icons/Lamp.png']);
      | end
  Lamp6 : Subsystem  DialogController=hmiCreateDDGDialog  IsWebBlock=on  mask(MWDashboardBlock){webBlockId=f963022c-aea4-457b-adfc-b083e719e9f5, webBlockType=lamp, ShowInLibBrowser=on, ShowInitialText=on, HMISrcModelName=spaceShuttleOriginal}
      mask prompts: webBlockType "WebBlock Type"; HMISrcModelName "Source Model"
      mask help: SimulinkHMI:dialogs:LampDialogDesc
      mask Help: helpview([docroot '/mapfiles/simulink.map'], 'hmi_lamp')
      mask Display:
      | if strcmp(get_param(bdroot(gcb),'BlockDiagramType'), 'library')
      |     image([(matlabroot) '/toolbox/simulink/hmi/icons/Lamp.png']);
      | end
  Lamp7 : Subsystem  DialogController=hmiCreateDDGDialog  IsWebBlock=on  mask(MWDashboardBlock){webBlockId=74668ae3-2b37-4bc0-806e-989ea60bf3f3, webBlockType=lamp, ShowInLibBrowser=on, ShowInitialText=on, HMISrcModelName=spaceShuttleOriginal}
      mask prompts: webBlockType "WebBlock Type"; HMISrcModelName "Source Model"
      mask help: SimulinkHMI:dialogs:LampDialogDesc
      mask Help: helpview([docroot '/mapfiles/simulink.map'], 'hmi_lamp')
      mask Display:
      | if strcmp(get_param(bdroot(gcb),'BlockDiagramType'), 'library')
      |     image([(matlabroot) '/toolbox/simulink/hmi/icons/Lamp.png']);
      | end
  Lamp8 : Subsystem  DialogController=hmiCreateDDGDialog  IsWebBlock=on  mask(MWDashboardBlock){webBlockId=a86ecc11-9b5f-486c-a116-6a169a848fb0, webBlockType=lamp, ShowInLibBrowser=on, ShowInitialText=on, HMISrcModelName=spaceShuttleOriginal}
      mask prompts: webBlockType "WebBlock Type"; HMISrcModelName "Source Model"
      mask help: SimulinkHMI:dialogs:LampDialogDesc
      mask Help: helpview([docroot '/mapfiles/simulink.map'], 'hmi_lamp')
      mask Display:
      | if strcmp(get_param(bdroot(gcb),'BlockDiagramType'), 'library')
      |     image([(matlabroot) '/toolbox/simulink/hmi/icons/Lamp.png']);
      | end
  Lamp9 : Subsystem  DialogController=hmiCreateDDGDialog  IsWebBlock=on  mask(MWDashboardBlock){webBlockId=f4dbbe1a-4ec4-452b-b5cc-403f6e1bd4d4, webBlockType=lamp, ShowInLibBrowser=on, ShowInitialText=on, HMISrcModelName=spaceShuttleOriginal}
      mask prompts: webBlockType "WebBlock Type"; HMISrcModelName "Source Model"
      mask help: SimulinkHMI:dialogs:LampDialogDesc
      mask Help: helpview([docroot '/mapfiles/simulink.map'], 'hmi_lamp')
      mask Display:
      | if strcmp(get_param(bdroot(gcb),'BlockDiagramType'), 'library')
      |     image([(matlabroot) '/toolbox/simulink/hmi/icons/Lamp.png']);
      | end
  Rotary Switch : Subsystem  DialogController=hmiCreateDDGDialog  IsWebBlock=on  mask(MWDashboardBlock){webBlockId=aad051ce-0605-48d0-815b-93b49174babb, webBlockType=discreteknob, ShowInLibBrowser=on, ShowInitialText=on, HMISrcModelName=spaceShuttleOriginal}
      mask prompts: webBlockId "WebBlock Id"; webBlockType "WebBlock Type"; HMISrcModelName "Source Model"
      mask help: SimulinkHMI:dialogs:DiscreteKnobDialogDesc
      mask Help: helpview([docroot '/mapfiles/simulink.map'], 'hmi_rotary_switch')
      mask Display:
      | model = bdroot(gcb);
      | if strcmp(get_param(model,'BlockDiagramType'), 'library')
      |     image([(matlabroot) '/toolbox/simulink/hmi/icons/DiscreteKnob.png']);
      | end
  Rotary Switch1 : Subsystem  DialogController=hmiCreateDDGDialog  IsWebBlock=on  mask(MWDashboardBlock){webBlockId=d0caed68-568e-4dc9-8d97-a2c88f43b8a4, webBlockType=discreteknob, ShowInLibBrowser=on, ShowInitialText=on, HMISrcModelName=spaceShuttleOriginal}
      mask prompts: webBlockId "WebBlock Id"; webBlockType "WebBlock Type"; HMISrcModelName "Source Model"
      mask help: SimulinkHMI:dialogs:DiscreteKnobDialogDesc
      mask Help: helpview([docroot '/mapfiles/simulink.map'], 'hmi_rotary_switch')
      mask Display:
      | model = bdroot(gcb);
      | if strcmp(get_param(model,'BlockDiagramType'), 'library')
      |     image([(matlabroot) '/toolbox/simulink/hmi/icons/DiscreteKnob.png']);
      | end
  Rotary Switch2 : Subsystem  DialogController=hmiCreateDDGDialog  IsWebBlock=on  mask(MWDashboardBlock){webBlockId=1c4c8ede-caaf-4351-9b32-2d96b9d3b069, webBlockType=discreteknob, ShowInLibBrowser=on, ShowInitialText=on, HMISrcModelName=spaceShuttleOriginal}
      mask prompts: webBlockId "WebBlock Id"; webBlockType "WebBlock Type"; HMISrcModelName "Source Model"
      mask help: SimulinkHMI:dialogs:DiscreteKnobDialogDesc
      mask Help: helpview([docroot '/mapfiles/simulink.map'], 'hmi_rotary_switch')
      mask Display:
      | model = bdroot(gcb);
      | if strcmp(get_param(model,'BlockDiagramType'), 'library')
      |     image([(matlabroot) '/toolbox/simulink/hmi/icons/DiscreteKnob.png']);
      | end
  Toggle Switch : Subsystem  DialogController=hmiCreateDDGDialog  IsWebBlock=on  mask(MWDashboardBlock){webBlockId=a1feb33e-c936-40cb-b89a-58db8a7ab2ae, webBlockType=toggleswitch, ShowInLibBrowser=on, ShowInitialText=on, HMISrcModelName=spaceShuttleOriginal}
      mask prompts: webBlockId "WebBlock Id"; webBlockType "WebBlock Type"; HMISrcModelName "Source Model"
      mask help: SimulinkHMI:dialogs:SwitchDialogDesc
      mask Help: helpview([docroot '/mapfiles/simulink.map'], 'hmi_toggle_switch')
      mask Display:
      | if strcmp(get_param(bdroot(gcb),'BlockDiagramType'), 'library')
      |     image([(matlabroot) '/toolbox/simulink/hmi/icons/ToggleSwitch.png']);
      | end
  Toggle Switch1 : Subsystem  DialogController=hmiCreateDDGDialog  IsWebBlock=on  mask(MWDashboardBlock){webBlockId=632d40ef-ab94-416f-9446-e5cd2c645a87, webBlockType=toggleswitch, ShowInLibBrowser=on, ShowInitialText=on, HMISrcModelName=spaceShuttleOriginal}
      mask prompts: webBlockId "WebBlock Id"; webBlockType "WebBlock Type"; HMISrcModelName "Source Model"
      mask help: SimulinkHMI:dialogs:SwitchDialogDesc
      mask Help: helpview([docroot '/mapfiles/simulink.map'], 'hmi_toggle_switch')
      mask Display:
      | if strcmp(get_param(bdroot(gcb),'BlockDiagramType'), 'library')
      |     image([(matlabroot) '/toolbox/simulink/hmi/icons/ToggleSwitch.png']);
      | end
  Toggle Switch2 : Subsystem  DialogController=hmiCreateDDGDialog  IsWebBlock=on  mask(MWDashboardBlock){webBlockId=c411ff4e-efdd-44a4-8e84-bf7aad950407, webBlockType=toggleswitch, ShowInLibBrowser=on, ShowInitialText=on, HMISrcModelName=spaceShuttleOriginal}
      mask prompts: webBlockId "WebBlock Id"; webBlockType "WebBlock Type"; HMISrcModelName "Source Model"
      mask help: SimulinkHMI:dialogs:SwitchDialogDesc
      mask Help: helpview([docroot '/mapfiles/simulink.map'], 'hmi_toggle_switch')
      mask Display:
      | if strcmp(get_param(bdroot(gcb),'BlockDiagramType'), 'library')
      |     image([(matlabroot) '/toolbox/simulink/hmi/icons/ToggleSwitch.png']);
      | end
  Toggle Switch3 : Subsystem  DialogController=hmiCreateDDGDialog  IsWebBlock=on  mask(MWDashboardBlock){webBlockId=72f03ffd-cacb-422d-91db-5f40b9d6549d, webBlockType=toggleswitch, ShowInLibBrowser=on, ShowInitialText=on, HMISrcModelName=spaceShuttleOriginal}
      mask prompts: webBlockId "WebBlock Id"; webBlockType "WebBlock Type"; HMISrcModelName "Source Model"
      mask help: SimulinkHMI:dialogs:SwitchDialogDesc
      mask Help: helpview([docroot '/mapfiles/simulink.map'], 'hmi_toggle_switch')
      mask Display:
      | if strcmp(get_param(bdroot(gcb),'BlockDiagramType'), 'library')
      |     image([(matlabroot) '/toolbox/simulink/hmi/icons/ToggleSwitch.png']);
      | end

== system spaceShuttleOriginal/Attitude Processing/SECOND_PASS == 0 ==
  x : Inport
  Action Port : ActionPort  ActionType=else
  Bus Assignment1 : BusAssignment  AssignedSignals=ATTITUDE_INCREMENT,CURRENT_ATTITUDE,ATTITUDE_ESTIMATE,RATE_ESTIMATE,UNDESIRED_ACCELERATION_ESTIMATE
  Constant2 : Constant
  Data Store Read : DataStoreRead  DataStoreName=ATTITUDE_INCREMENT
  Data Store Read1 : DataStoreRead  DataStoreName=CURRENT_ATTITUDE
  Data Store Read2 : DataStoreRead  DataStoreName=RATE_ESTIMATE
  Data Store Read3 : DataStoreRead  DataStoreName=ATTITUDE_ESTIMATE
  Data Store Read4 : DataStoreRead  DataStoreName=UNDESIRED_ACCELERATION_ESTIMATE
  Data Store Write1 : DataStoreWrite  DataStoreName=SECOND_PASS
  y : Outport
  wires:
  Constant2/1 -> Data Store Write1/1
  x/1 -> Bus Assignment1/1
  Bus Assignment1/1 -> y/1
  Data Store Read/1 -> Bus Assignment1/2
  Data Store Read1/1 -> Bus Assignment1/3
  Data Store Read3/1 -> Bus Assignment1/4
  Data Store Read2/1 -> Bus Assignment1/5
  Data Store Read4/1 -> Bus Assignment1/6

== system spaceShuttleOriginal/Attitude Processing/SECOND_PASS == 1 ==
  x : Inport
  R_I_B : Inport  Port=2
  R_I_B1 : Inport  Port=3
  Action Port : ActionPort  ActionType=then
  ATTITUDE PROCESSOR : Subsystem
  Bus Assignment : BusAssignment  AssignedSignals=ATTITUDE_INCREMENT,CURRENT_ATTITUDE,ATTITUDE_ESTIMATE,RATE_ESTIMATE,UNDESIRED_ACCELERATION_ESTIMATE
  Constant2 : Constant  Value=0
  Data Store Write1 : DataStoreWrite  DataStoreName=SECOND_PASS
  Data Store Write2 : DataStoreWrite  DataStoreName=CURRENT_ATTITUDE
  Data Store Write3 : DataStoreWrite  DataStoreName=ATTITUDE_INCREMENT
  Data Store Write4 : DataStoreWrite  DataStoreName=ATTITUDE_ESTIMATE
  Data Store Write5 : DataStoreWrite  DataStoreName=RATE_ESTIMATE
  Data Store Write6 : DataStoreWrite  DataStoreName=UNDESIRED_ACCELERATION_ESTIMATE
  State Estimator Part I : Subsystem
  y : Outport
  wires:
  Bus Assignment/1 -> y/1
  Constant2/1 -> Data Store Write1/1
  ATTITUDE PROCESSOR/1(CURRENT ATTITUDE) -> State Estimator Part I/1(CURRENT_ATTITUDE), Bus Assignment/3, Data Store Write2/1
  ATTITUDE PROCESSOR/2(ATTITUDE INCREMENT) -> Bus Assignment/2, Data Store Write3/1
  R_I_B/1 -> ATTITUDE PROCESSOR/1(R_I_B)
  R_I_B1/1 -> ATTITUDE PROCESSOR/2(R_I_B_PREVIOUS)
  x/1 -> Bus Assignment/1
  State Estimator Part I/1(ATTITUDE_ESTIMATE) -> Bus Assignment/4, Data Store Write4/1
  State Estimator Part I/2(RATE_ESTIMATE) -> Bus Assignment/5, Data Store Write5/1
  State Estimator Part I/3(UNDESIRED_ACCELERATION_ESTIMATE) -> Bus Assignment/6, Data Store Write6/1

== system spaceShuttleOriginal/Auto // Manual Maneuver/IF MANUAL ==
  x : Inport
  Action Port : ActionPort  ActionType=else
  MANUAL MANEUVER MODULE : Subsystem
  y : Outport
  wires:
  x/1 -> MANUAL MANEUVER MODULE/1(In1)
  MANUAL MANEUVER MODULE/1(Out1) -> y/1

== system spaceShuttleOriginal/Auto // Manual Maneuver/If AUTO ==
  x : Inport
  Action Port : ActionPort  ActionType=then
  Bus Selector1 : BusSelector  OutputSignals=AUTO_MANUAL_SWITCH
  Bus Selector2 : BusSelector  OutputSignals=COUNTER
  COUNTER ~=0 : Subsystem  TreatAsAtomicUnit=on
  IF COUNTER=0 : Subsystem  TreatAsAtomicUnit=on
  IF OLD=AUTO : Subsystem  TreatAsAtomicUnit=on
  IF OLD=MANUAL : Subsystem  TreatAsAtomicUnit=on
  If : If  IfExpression=u1 == 0
  If1 : If  IfExpression=u1 == 0
  Merge : Merge
  Merge1 : Merge
  Selector : Selector  InputPortWidth=2  IndexOptions=Index vector (dialog)  Indices=[2]  OutputSizes=1
  Out1 : Outport
  wires:
  Bus Selector1/1 -> Selector/1  "<AUTO_MANUAL_SWITCH>"
  If/1 -> IF OLD=MANUAL/Action
  x/1 -> IF OLD=AUTO/1(In1), IF OLD=MANUAL/1(In1), Bus Selector1/1
  Merge/1 -> IF COUNTER=0/1(In2), COUNTER ~=0/1(In1), Bus Selector2/1
  If1/1 -> IF COUNTER=0/Action
  IF OLD=MANUAL/1(Out1) -> Merge/1
  IF OLD=AUTO/1(Out1) -> Merge/2
  If/2 -> IF OLD=AUTO/Action
  If1/2 -> COUNTER ~=0/Action
  COUNTER ~=0/1(Out1) -> Merge1/2
  Bus Selector2/1 -> If1/1  "<COUNTER>"
  Merge1/1 -> Out1/1
  IF COUNTER=0/1(Out1) -> Merge1/1
  Selector/1 -> If/1

== system spaceShuttleOriginal/Call Jet Select/PRIMARY JETS ==
  In1 : Inport
  Action Port : ActionPort  ActionType=then
  Bus Assignment : BusAssignment  AssignedSignals=PRIMARY_JET_COMMAND,VERNIER_JET_COMMAND
  Bus Selector : BusSelector  OutputSignals=ROTATION_COMMAND,USER_INPUTS.PITCH_HI_LOW_SW,USER_INPUTS.NO_PLUS_Z_JETS,USER_INPUTS.PITCH_TAIL_NOSE_SW,USER_INPUTS.YAW_HI_LOW_SW,USER_INPUTS.YAW_TAIL_NOSE_SW
  Constant{,1..3} (4 alike) : Constant  Value=0
  Data Store Write : DataStoreWrite  DataStoreName=PRIMARY_JET_COMMAND
  Data Store Write1 : DataStoreWrite  DataStoreName=VERNIER_JET_COMMAND
  MATLAB Function : MATLAB Function  TreatAsAtomicUnit=on
  Mux : Mux  Inputs=3
  Mux1 : Mux  Inputs=6
  y : Outport
  wires:
  Bus Selector/4 -> MATLAB Function/5(PITCH_TAIL_NOSE_SW)  "<PITCH_TAIL_NOSE_SW>"
  Mux/1 -> MATLAB Function/1(compensationCommand)
  Bus Selector/5 -> MATLAB Function/6(YAW_HI_LOW_SW)  "<YAW_HI_LOW_SW>"
  Bus Selector/6 -> MATLAB Function/7(YAW_TAIL_NOSE_SW)  "<YAW_TAIL_NOSE_SW>"
  Bus Selector/3 -> MATLAB Function/4(NO_PLUS_Z_JETS)  "<NO_PLUS_Z_JETS>"
  Bus Selector/1 -> MATLAB Function/2(rotationCommand)  "<ROTATION_COMMAND>"
  In1/1 -> Bus Selector/1, Bus Assignment/1
  MATLAB Function/1(primaryJetCommand) -> Bus Assignment/2, Data Store Write/1
  Constant2/1 -> Mux/3
  Bus Selector/2 -> MATLAB Function/3(PITCH_HI_LOW_SW)  "<PITCH_HI_LOW_SW>"
  Bus Assignment/1 -> y/1
  Constant1/1 -> Mux/2
  Constant/1 -> Mux/1
  Constant3/1 -> Mux1/6, Mux1/5, Mux1/4, Mux1/1, Mux1/2, Mux1/3
  Mux1/1 -> Bus Assignment/3, Data Store Write1/1

== system spaceShuttleOriginal/Call Jet Select/VERNIER JETS ==
  x : Inport
  Action Port : ActionPort  ActionType=else
  Bus Assignment : BusAssignment  AssignedSignals=VERNIER_JET_COMMAND,PRIMARY_JET_COMMAND
  Constant : Constant  Value=0
  Data Store Write : DataStoreWrite  DataStoreName=PRIMARY_JET_COMMAND
  Data Store Write1 : DataStoreWrite  DataStoreName=VERNIER_JET_COMMAND
  MATLAB Function : MATLAB Function  TreatAsAtomicUnit=on
  Mux : Mux  Inputs=11
  y : Outport
  wires:
  Bus Assignment/1 -> y/1
  Mux/1 -> Bus Assignment/3, Data Store Write/1
  x/1 -> Bus Assignment/1
  Constant/1 -> Mux/2, Mux/1, Mux/3, Mux/4, Mux/5, Mux/11, Mux/10, Mux/9, Mux/8, Mux/7, Mux/6
  MATLAB Function/1(vernierJetCommand) -> Bus Assignment/2, Data Store Write1/1

== system spaceShuttleOriginal/Call Phase Plane/Get Rotation Pitch ==
  In1 : Inport
  Bus Selector : BusSelector  OutputSignals=USER_INPUTS.PRIMARY_VERNIER_SW,UNDESIRED_ACCELERATION_ESTIMATE,USER_INPUTS.DEADBAND,ATTITUDE_ERROR,RATE_ERROR,ROTATION_COMMAND,USER_INPUTS.RATE_LIMIT,BYPASS,FORCE_FIRE
  Constant : Constant  Value=2
  Constant1 : Constant  Value=2
  Constant2 : Constant  Value=2
  Display1 : Display
  MATLAB Function : MATLAB Function  TreatAsAtomicUnit=on
  MATLAB Function1 : MATLAB Function  TreatAsAtomicUnit=on
  MATLAB Function2 : MATLAB Function  TreatAsAtomicUnit=on
  Out1 : Outport
  wires:
  MATLAB Function2/1(command) -> Out1/1
  Constant/1 -> MATLAB Function/1(n)
  MATLAB Function/1(S) -> MATLAB Function1/2(S), MATLAB Function2/3(S)
  Bus Selector/8 -> MATLAB Function2/5(BYPASS)  "<BYPASS>"
  MATLAB Function1/1(index) -> Display1/1, MATLAB Function2/2(index)
  Constant1/1 -> MATLAB Function2/1(n)
  Bus Selector/9 -> MATLAB Function2/9(forceFire)  "<FORCE_FIRE>"
  Constant2/1 -> MATLAB Function1/1(n)
  Bus Selector/7 -> MATLAB Function2/8(rateLimit), MATLAB Function/8(rateLimit)  "<RATE_LIMIT>"
  In1/1 -> Bus Selector/1
  Bus Selector/6 -> MATLAB Function2/6(RC), MATLAB Function/7(rotationCommandn)  "<ROTATION_COMMAND>"
  Bus Selector/5 -> MATLAB Function1/4(we), MATLAB Function2/7(rate_error), MATLAB Function/6(rate_error)  "<RATE_ERROR>"
  Bus Selector/4 -> MATLAB Function1/3(theta_e), MATLAB Function/5(attitude_error)  "<ATTITUDE_ERROR>"
  Bus Selector/3 -> MATLAB Function/4(DB)  "<DEADBAND>"
  Bus Selector/2 -> MATLAB Function1/5(undesired_acc), MATLAB Function/3(undesired_acc)  "<UNDESIRED_ACCELERATION_ESTIMATE>"
  Bus Selector/1 -> MATLAB Function2/4(vernier_sw), MATLAB Function/2(vernier_sw)  "<PRIMARY_VERNIER_SW>"

== system spaceShuttleOriginal/Call Phase Plane/Get Rotation Roll ==
  In1 : Inport
  Bus Selector : BusSelector  OutputSignals=USER_INPUTS.PRIMARY_VERNIER_SW,UNDESIRED_ACCELERATION_ESTIMATE,USER_INPUTS.DEADBAND,ATTITUDE_ERROR,RATE_ERROR,ROTATION_COMMAND,USER_INPUTS.RATE_LIMIT,BYPASS,FORCE_FIRE
  Constant : Constant
  Constant1 : Constant
  Constant2 : Constant
  Display1 : Display
  MATLAB Function : MATLAB Function  TreatAsAtomicUnit=on
  MATLAB Function1 : MATLAB Function  TreatAsAtomicUnit=on
  MATLAB Function2 : MATLAB Function  TreatAsAtomicUnit=on
  Out1 : Outport
  wires:
  MATLAB Function2/1(command) -> Out1/1
  Constant/1 -> MATLAB Function/1(n)
  MATLAB Function/1(S) -> MATLAB Function1/2(S), MATLAB Function2/3(S)
  Bus Selector/8 -> MATLAB Function2/5(BYPASS)  "<BYPASS>"
  MATLAB Function1/1(index) -> Display1/1, MATLAB Function2/2(index)
  Constant1/1 -> MATLAB Function2/1(n)
  Bus Selector/9 -> MATLAB Function2/9(forceFire)  "<FORCE_FIRE>"
  Constant2/1 -> MATLAB Function1/1(n)
  Bus Selector/7 -> MATLAB Function2/8(rateLimit), MATLAB Function/8(rateLimit)  "<RATE_LIMIT>"
  In1/1 -> Bus Selector/1
  Bus Selector/6 -> MATLAB Function2/6(RC), MATLAB Function/7(rotationCommandn)  "<ROTATION_COMMAND>"
  Bus Selector/5 -> MATLAB Function1/4(we), MATLAB Function2/7(rate_error), MATLAB Function/6(rate_error)  "<RATE_ERROR>"
  Bus Selector/4 -> MATLAB Function1/3(theta_e), MATLAB Function/5(attitude_error)  "<ATTITUDE_ERROR>"
  Bus Selector/3 -> MATLAB Function/4(DB)  "<DEADBAND>"
  Bus Selector/2 -> MATLAB Function1/5(undesired_acc), MATLAB Function/3(undesired_acc)  "<UNDESIRED_ACCELERATION_ESTIMATE>"
  Bus Selector/1 -> MATLAB Function2/4(vernier_sw), MATLAB Function/2(vernier_sw)  "<PRIMARY_VERNIER_SW>"

== system spaceShuttleOriginal/Call Phase Plane/Get Rotation Yaw ==
  In1 : Inport
  Bus Selector : BusSelector  OutputSignals=USER_INPUTS.PRIMARY_VERNIER_SW,UNDESIRED_ACCELERATION_ESTIMATE,USER_INPUTS.DEADBAND,ATTITUDE_ERROR,RATE_ERROR,ROTATION_COMMAND,USER_INPUTS.RATE_LIMIT,BYPASS,FORCE_FIRE
  Constant : Constant  Value=3
  Constant1 : Constant  Value=3
  Constant2 : Constant  Value=3
  Display1 : Display
  MATLAB Function : MATLAB Function  TreatAsAtomicUnit=on
  MATLAB Function1 : MATLAB Function  TreatAsAtomicUnit=on
  MATLAB Function2 : MATLAB Function  TreatAsAtomicUnit=on
  Out1 : Outport
  wires:
  MATLAB Function2/1(command) -> Out1/1
  Constant/1 -> MATLAB Function/1(n)
  MATLAB Function/1(S) -> MATLAB Function1/2(S), MATLAB Function2/3(S)
  Bus Selector/8 -> MATLAB Function2/5(BYPASS)  "<BYPASS>"
  MATLAB Function1/1(index) -> Display1/1, MATLAB Function2/2(index)
  Constant1/1 -> MATLAB Function2/1(n)
  Bus Selector/9 -> MATLAB Function2/9(forceFire)  "<FORCE_FIRE>"
  Constant2/1 -> MATLAB Function1/1(n)
  Bus Selector/7 -> MATLAB Function2/8(rateLimit), MATLAB Function/8(rateLimit)  "<RATE_LIMIT>"
  In1/1 -> Bus Selector/1
  Bus Selector/6 -> MATLAB Function2/6(RC), MATLAB Function/7(rotationCommandn)  "<ROTATION_COMMAND>"
  Bus Selector/5 -> MATLAB Function1/4(we), MATLAB Function2/7(rate_error), MATLAB Function/6(rate_error)  "<RATE_ERROR>"
  Bus Selector/4 -> MATLAB Function1/3(theta_e), MATLAB Function/5(attitude_error)  "<ATTITUDE_ERROR>"
  Bus Selector/3 -> MATLAB Function/4(DB)  "<DEADBAND>"
  Bus Selector/2 -> MATLAB Function1/5(undesired_acc), MATLAB Function/3(undesired_acc)  "<UNDESIRED_ACCELERATION_ESTIMATE>"
  Bus Selector/1 -> MATLAB Function2/4(vernier_sw), MATLAB Function/2(vernier_sw)  "<PRIMARY_VERNIER_SW>"

== system spaceShuttleOriginal/First Pass/If First Pass ==
  In1 : Inport
  Action Port : ActionPort  ActionType=then
  AUTO : Subsystem  TreatAsAtomicUnit=on
  Bus Assignment : BusAssignment  AssignedSignals=INIT_JET_SELECT
  Bus Selector : BusSelector  OutputSignals=AUTO_MANUAL_SWITCH
  Constant2 : Constant
  Data Store Write1 : DataStoreWrite  DataStoreName=INIT_JET_SELECT
  If : If  IfExpression=u1 == 0
  MANUAL : Subsystem  TreatAsAtomicUnit=on
  Merge : Merge
  Selector : Selector  InputPortWidth=2  IndexOptions=Index vector (dialog)  Indices=[1]  OutputSizes=1
  x : Outport
  wires:
  In1/1 -> Bus Assignment/1
  Bus Assignment/1 -> AUTO/1(In2), MANUAL/1(In1), Bus Selector/1
  Constant2/1 -> Bus Assignment/2, Data Store Write1/1
  Bus Selector/1 -> Selector/1  "<AUTO_MANUAL_SWITCH>"
  If/1 -> MANUAL/Action
  If/2 -> AUTO/Action
  MANUAL/1(x) -> Merge/1
  Merge/1 -> x/1
  Selector/1 -> If/1
  AUTO/1(x1) -> Merge/2

== system spaceShuttleOriginal/First Pass/If not first pass ==
  In1 : Inport
  Action Port : ActionPort  ActionType=else
  Bus Assignment : BusAssignment  AssignedSignals=INIT_JET_SELECT,INIT_STATE_ERROR
  Data Store Read : DataStoreRead  DataStoreName=INIT_JET_SELECT
  Data Store Read1 : DataStoreRead  DataStoreName=INIT_STATE_ERROR
  x : Outport
  wires:
  In1/1 -> Bus Assignment/1
  Data Store Read/1 -> Bus Assignment/2
  Bus Assignment/1 -> x/1
  Data Store Read1/1 -> Bus Assignment/3

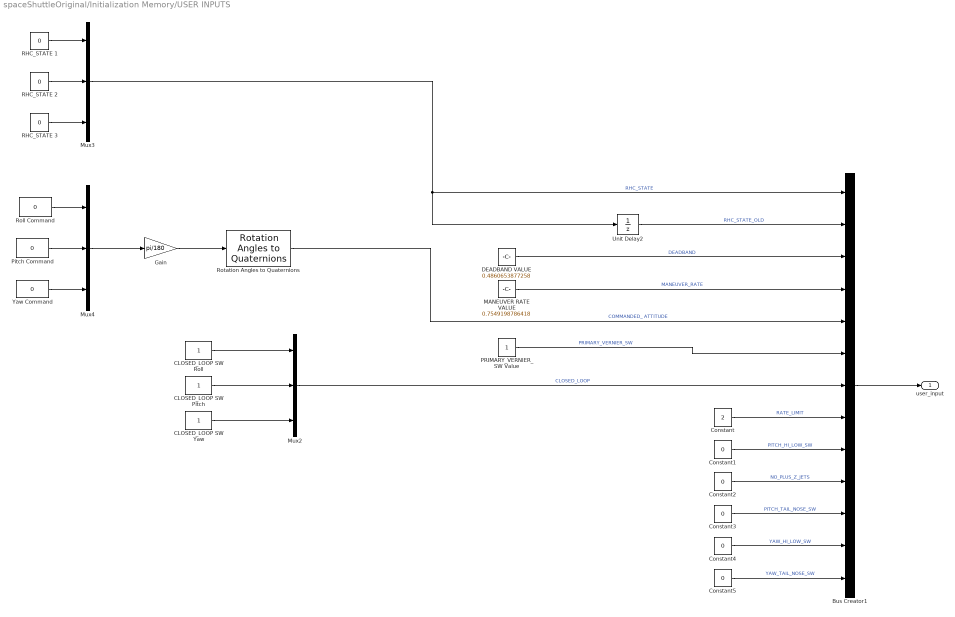
== system spaceShuttleOriginal/Initialization Memory/USER INPUTS ==
  Bus Creator1 : BusCreator  Inputs=13
  CLOSED_LOOP SW Pitch : Constant
  CLOSED_LOOP SW Roll : Constant
  CLOSED_LOOP SW Yaw : Constant
  Constant : Constant  Value=2
  Constant{1..5} (5 alike) : Constant  Value=0
  DEADBAND VALUE : Constant  Value=0.4860653877258
  Gain : Gain  Gain=pi/180
  MANEUVER RATE VALUE : Constant  Value=0.7549198786418
  Mux2 : Mux  Inputs=3
  Mux3 : Mux  Inputs=3
  Mux4 : Mux  Inputs=3
  PRIMARY_VERNIER_SW Value : Constant
  Pitch Command : Constant  Value=0
  RHC_STATE 1 : Constant  Value=0
  RHC_STATE 2 : Constant  Value=0
  RHC_STATE 3 : Constant  Value=0
  Roll Command : Constant  Value=0
  Rotation Angles to Quaternions : sharedtransform/Rotation Angles to Quaternions  rotationOrder=XYZ
      settings: SourceProductName=Aerospace Blockset  SourceProductBaseCode=AE
  Unit Delay2 : UnitDelay  SampleTime=-1
  Yaw Command : Constant  Value=0
  user_input : Outport
  wires:
  RHC_STATE 1/1 -> Mux3/1
  RHC_STATE 3/1 -> Mux3/3
  DEADBAND VALUE/1 -> Bus Creator1/3  "DEADBAND"
  MANEUVER RATE VALUE/1 -> Bus Creator1/4  "MANEUVER_RATE"
  Rotation Angles to Quaternions/1 -> Bus Creator1/5  "COMMANDED_ ATTITUDE"
  Mux2/1 -> Bus Creator1/7  "CLOSED_LOOP"
  CLOSED_LOOP SW Roll/1 -> Mux2/1
  CLOSED_LOOP SW Pitch/1 -> Mux2/2
  CLOSED_LOOP SW Yaw/1 -> Mux2/3
  RHC_STATE 2/1 -> Mux3/2
  Constant/1 -> Bus Creator1/8  "RATE_LIMIT"
  Constant1/1 -> Bus Creator1/9  "PITCH_HI_LOW_SW"
  Constant2/1 -> Bus Creator1/10  "NO_PLUS_Z_JETS"
  Constant3/1 -> Bus Creator1/11  "PITCH_TAIL_NOSE_SW"
  Constant4/1 -> Bus Creator1/12  "YAW_HI_LOW_SW"
  Constant5/1 -> Bus Creator1/13  "YAW_TAIL_NOSE_SW"
  Mux3/1 -> Unit Delay2/1, Bus Creator1/1  "RHC_STATE"
  Yaw Command/1 -> Mux4/3
  Pitch Command/1 -> Mux4/2
  Roll Command/1 -> Mux4/1
  Mux4/1 -> Gain/1
  Gain/1 -> Rotation Angles to Quaternions/1
  PRIMARY_VERNIER_SW Value/1 -> Bus Creator1/6  "PRIMARY_VERNIER_SW"
  Unit Delay2/1 -> Bus Creator1/2  "RHC_STATE_OLD"
  Bus Creator1/1 -> user_input/1

== system spaceShuttleOriginal/State Error/Coordinate 1 ==
  In1 : Inport
  Bus Selector : BusSelector  OutputSignals=INIT_STATE_ERROR
  INIT STATE ERROR = OFF : Subsystem  TreatAsAtomicUnit=on
  INIT STATE ERROR = ON : Subsystem  TreatAsAtomicUnit=on
  If : If  IfExpression=u1 == 1
  Merge : Merge
  Selector : Selector  InputPortWidth=3  IndexOptions=Index vector (dialog)  Indices=[1]  OutputSizes=1
  y : Outport
  wires:
  In1/1 -> INIT STATE ERROR = OFF/1(In1), INIT STATE ERROR = ON/1(In1), Bus Selector/1
  Bus Selector/1 -> Selector/1  "<INIT_STATE_ERROR>"
  If/2 -> INIT STATE ERROR = OFF/Action
  Selector/1 -> If/1
  If/1 -> INIT STATE ERROR = ON/Action
  Merge/1 -> y/1
  INIT STATE ERROR = ON/1(y) -> Merge/1
  INIT STATE ERROR = OFF/1(y1) -> Merge/2
